simulink model "nz"  (R2018a)
settings: Solver=VariableStepAuto  StartTime=0.0  StopTime=10.0  RelTol=1e-3
settings Model: Creator=master  LastModifiedBy=master

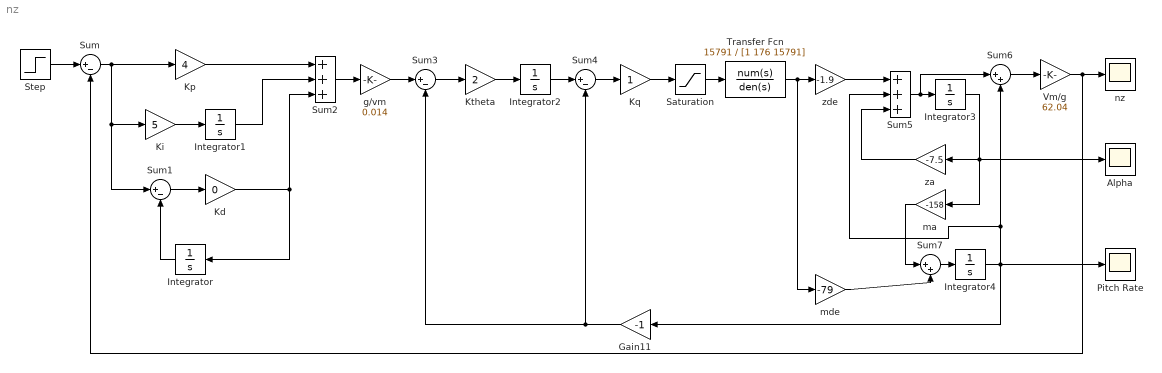
== system nz ==
  Alpha : Scope
  Gain11 : Gain  Gain=-1
  Integrator{,1..4} (5 alike) : Integrator
  Kd : Gain  Gain=0
  Ki : Gain  Gain=5
  Kp : Gain  Gain=4
  Kq : Gain
  Ktheta : Gain  Gain=2
  Pitch Rate : Scope
  Saturation : Saturate  UpperLimit=0.35  LowerLimit=-0.35
  Step : Step  SampleTime=0
  Sum{,1,3..4} (4 alike) : Sum  Inputs=|+-
  Sum2 : Sum  Inputs=+++
  Sum5 : Sum  Inputs=+++
  Sum6 : Sum  Inputs=|++
  Sum7 : Sum  Inputs=|++
  Transfer Fcn : TransferFcn  Numerator=15791  Denominator=[1 176 15791]
  Vm/g : Gain  Gain=62.04
  g/vm : Gain  Gain=0.014
  ma : Gain  Gain=-158
  mde : Gain  Gain=-79
  nz : Scope
  za : Gain  Gain=-7.5
  zde : Gain  Gain=-1.9
  wires:
  Sum1/1 -> Kd/1
  Integrator/1 -> Sum1/2
  Sum/1 -> Sum1/1, Ki/1, Kp/1
  Kp/1 -> Sum2/1
  Sum2/1 -> g/vm/1
  Ki/1 -> Integrator1/1
  Integrator1/1 -> Sum2/2
  Kd/1 -> Integrator/1, Sum2/3
  Step/1 -> Sum/1
  g/vm/1 -> Sum3/1
  Sum3/1 -> Ktheta/1
  Ktheta/1 -> Integrator2/1
  Integrator2/1 -> Sum4/1
  Sum4/1 -> Kq/1
  Kq/1 -> Saturation/1
  Saturation/1 -> Transfer Fcn/1
  Transfer Fcn/1 -> mde/1, zde/1
  zde/1 -> Sum5/1
  Sum5/1 -> Sum6/1, Integrator3/1
  Sum6/1 -> Vm/g/1
  Vm/g/1 -> Sum/2, nz/1
  Integrator3/1 -> Alpha/1, za/1, ma/1
  ma/1 -> Sum7/1
  Sum7/1 -> Integrator4/1
  Integrator4/1 -> Gain11/1, Pitch Rate/1, Sum6/2, Sum5/2
  za/1 -> Sum5/3
  mde/1 -> Sum7/2
  Gain11/1 -> Sum3/2, Sum4/2
